simulink model "asservissement_vis_sans_fin_test"  (R2019a)
settings: Solver=VariableStepAuto  StartTime=0.0  StopTime=600000  RelTol=1e-3
model workspace (MAT data in the model file):
  Cx = 0.84
  S = 0.005625
libraries: fl_lib x14, nesl_utility x7, ee_lib x4, shared3dof x1, simulink x1, dspswit3 x1, sdl_lib x1
settings Model: Creator=Paul  LastModifiedBy=Paul

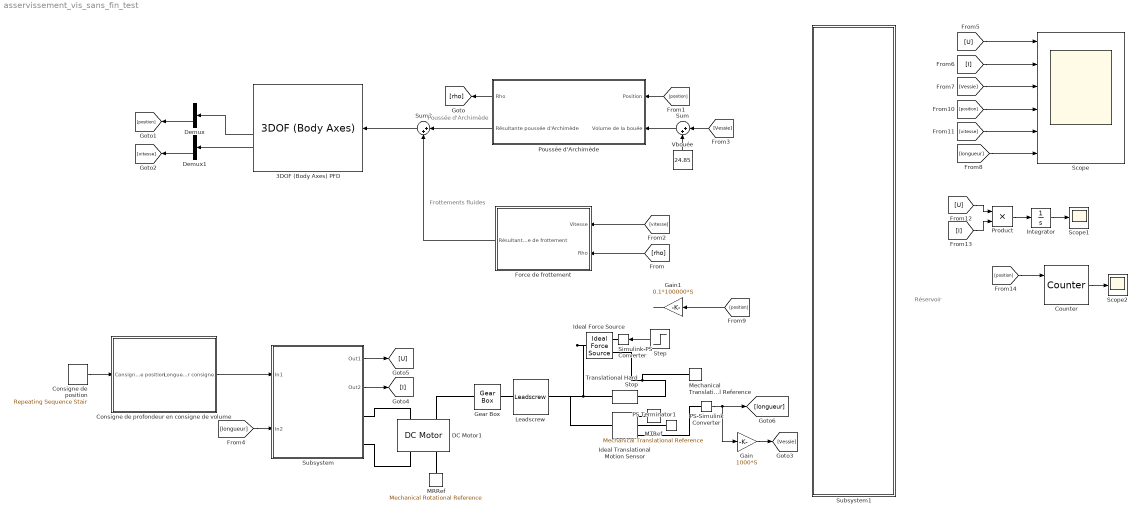
== system asservissement_vis_sans_fin_test ==
  note: Poussée d'Archimède
  note: Réservoir
  note: Frottements fluides
  "3DOF (Body Axes) PFD " : shared3dof/3DOF (Body Axes)  units=Metric (MKS)  mtype=Fixed  v_ini=0  theta_ini=0  alpha_ini=0  pos_ini=[0 0]  q_ini=0  mass=26  mass_e=0.5  mass_f=3.0  Iyy=1.0  Iyy_e=0.5  Iyy_f=3.0  g_in=Internal  g=9.81  vre_flag=on  abi_flag=off  aMode=0  vel_statename=''  theta_statename=''  pos_statename=''  q_statename=''  mass_statename=''
      settings: SourceProductName=Aerospace Blockset  SourceProductBaseCode=AE
  "Consigne de position " : simulink/Sources/Repeating Sequence Stair  OutValues=[0 1000 1000 1000 4000 0].'  tsamp=100000  OutMin=[]  OutMax=[]  OutDataTypeStr=double  OutputDataTypeScalingMode=double  OutDataType=fixdt(0,8)  ConRadixGroup=Best Precision: Vector-wise  OutScaling=2^-12
  Consigne de profondeur en consigne de volume : Subsystem
  Counter : dspswit3/Counter  Direction=Up  CountEvent=Falling edge  CounterSize=User defined  MaxCount=255  InitialCount=0  Output=Count  HitValue=32  ResetInput=on  SamplesPerFrame=1  Ts=1  CntDtype=double  HitDtype=Logical
  DC Motor1 : ee_lib/Electromechanical/Brushed Motors/DC Motor  parameterization=3  Ra=10 Ohm  La=0.0001 H  emf_or_torque=1  Kv=0.1 V/rpm  Ki=6.876e-4 N*m/A  T_stall=0.24e-3 N*m  w_max=5000 rpm  w_rated=4000 rpm  P_rated=400 W  V_rated=12 V  J=2000 g*cm^2  lam_param=1  lam=1e-6 N*m/(rad/s)  i_noload=0 A  V_i_noload=1.5 V  speed0=0 rpm  alpha=3.93e-3 1/K  Tmeas=25 degC  thermal_mass=100 J/K  initial_temperature=25 degC
      settings: SourceProductName=Simscape Electrical
  Demux : Demux  Outputs=2
  Demux1 : Demux  Outputs=2
  Force de frottement : Subsystem
  Gain : Gain  Gain=1000*S
  Gain1 : Gain  Gain=0.1*100000*S
  Gear Box : fl_lib/Mechanical/Mechanisms/Gear Box  ratio=50  t_in_specify=off  t_in_priority=None  t_in=0 N*m  t_in_nominal_specify=off  t_in_nominal_unit=N*m  t_in_nominal_value=1  t_out_specify=off  t_out_priority=None  t_out=0 N*m  t_out_nominal_specify=off  t_out_nominal_unit=N*m  t_out_nominal_value=1
  Ideal Force Source : fl_lib/Mechanical/Mechanical Sources/Ideal Force Source
  Ideal Translational Motion Sensor : fl_lib/Mechanical/Mechanical Sensors/Ideal Translational Motion Sensor  Tag=Factory Generic  offset=0.08 m
  Integrator : Integrator
  Leadscrew : sdl_lib/Gears/Rotational- Translational/Leadscrew  Lead=0.015 m  helix_type=1  friction_model=2  friction_parameterization=2  lambda=15 deg  alpha=14.5 deg  fr_coeff=0.08  eff_sn=0.9  eff_ns=0  mu_visc=0 N*m/(rad/s)  pwr_thr=0.001 W  temperature_TLU=[280, 300, 320] K  efficiency_sn_TLU=[.75, .65, .6]  efficiency_ns_TLU=[.5, .45, .4]  thermal_mass=50 J/K  T_init=300 K
      settings: SourceProductName=Simscape Driveline  SourceProductBaseCode=LD
  MRRef : fl_lib/Mechanical/Rotational Elements/Mechanical Rotational Reference
  MTRef : fl_lib/Mechanical/Translational Elements/Mechanical Translational Reference  Tag=Factory Generic
  Mechanical Translational Reference : fl_lib/Mechanical/Translational Elements/Mechanical Translational Reference
  PS Terminator1 : fl_lib/Physical Signals/Sinks/PS Terminator
      settings: SourceProductName=Simscape
  PS-Simulink Converter : nesl_utility/PS-Simulink Converter  PhysicalDomain=network_engine_domain  SubClassName=ps_output  LeftPortType=input  RightPortType=output  PseudoPeriodic=off  Frequencies=[]  Unit=1  AffineConversion=off
  Poussée d'Archimède : Subsystem
  Product : Product
  Scope : Scope  NumInputPorts=6
  Scope1 : Scope
  Scope2 : Scope
  Simulink-PS Converter : nesl_utility/Simulink-PS Converter  PhysicalDomain=network_engine_domain  SubClassName=ps_input  LeftPortType=input  RightPortType=output  PseudoPeriodic=off  Frequencies=[]  NoiseDistribution=none  NoiseParameters=[]  Unit=N  AffineConversion=off  FilteringAndDerivatives=provide  SimscapeFilterOrder=1  InputFilterTimeConstant=0.001  UdotUserProvided=0
  Step : Step  Time=490000  After=0  SampleTime=0
  Subsystem : Subsystem
  Subsystem1 : Subsystem
      mask Display: image('D:\Paul\Documents\TIPE\matlab\Les+flotteurs+Argo2.jpg');
  Sum : Sum  Inputs=|++
  Sum3 : Sum  Inputs=|++
  Translational Hard Stop : fl_lib/Mechanical/Translational Elements/Translational Hard Stop  upper_bnd=0.1 m  lower_bnd=-0.1 m  stiff_up=1e6 N/m  stiff_low=1e6 N/m  D_up=150 N/(m/s)  D_low=150 N/(m/s)  model=simscape.enum.hardstop.smooth  transition=0.1 mm  v_specify=off  v_priority=None  v=0 m/s  v_nominal_specify=off  v_nominal_unit=m/s  v_nominal_value=1  f_specify=off  f_priority=None  f=0 N  f_nominal_specify=off  f_nominal_unit=N  f_nominal_value=1  x_specify=off  x_priority=High  x=0 m  x_nominal_specify=off  x_nominal_unit=m  x_nominal_value=1
  Vbouée : Constant  Value=24.85
  wires:
  Force de frottement/1(Résultante force de frottement) -> Sum3/2
  [rho] -> Force de frottement/2(Rho)
  [U] -> Product/1
  Vbouée/1 -> Sum/2
  [position] -> Scope/4
  Demux/2 -> [position]
  [Vessie] -> Sum/1
  [I] -> Scope/2
  "3DOF (Body Axes) PFD "/5 -> Demux1/1
  "3DOF (Body Axes) PFD "/4 -> Demux/1
  [vitesse] -> Scope/5
  Demux1/2 -> [vitesse]
  Product/1 -> Integrator/1
  Poussée d'Archimède/2(Résultante poussée d'Archimède) -> Sum3/1
  [vitesse] -> Force de frottement/1(Vitesse)
  [Vessie] -> Scope/3
  [position] -> Counter/1
  [U] -> Scope/1
  Poussée d'Archimède/1("Rho ") -> [rho]
  [position] -> Poussée d'Archimède/1(Position)
  Integrator/1 -> Scope1/1
  Sum3/1 -> "3DOF (Body Axes) PFD "/2
  [I] -> Product/2
  Sum/1 -> Poussée d'Archimède/2(Volume de la bouée)
  Counter/1 -> Scope2/1
  PS-Simulink Converter/1 -> [longueur], Gain/1
  Consigne de profondeur en consigne de volume/1(Longueur consigne) -> Subsystem/1(In1)
  "Consigne de position "/1 -> Consigne de profondeur en consigne de volume/1(Consigne de position)
  Gain/1 -> [Vessie]
  [longueur] -> Subsystem/2(In2)
  Subsystem/1(Out1) -> [U]
  Subsystem/2(Out2) -> [I]
  [longueur] -> Scope/6
  Gain1/1 -> ?
  [position] -> Gain1/1
  Step/1 -> Simulink-PS Converter/1
  connections:
  DC Motor1/RConn2 -- MRRef/LConn1
  Gear Box/RConn1 -- Leadscrew/LConn1
  Gear Box/LConn1 -- DC Motor1/LConn2
  Ideal Force Source/LConn1 -- Translational Hard Stop/LConn1 -- Leadscrew/RConn1 -- Ideal Translational Motion Sensor/LConn1
  DC Motor1/LConn1 -- Subsystem/RConn1
  DC Motor1/RConn1 -- Subsystem/RConn2
  Ideal Force Source/RConn2 -- Translational Hard Stop/RConn1 -- Mechanical Translational Reference/LConn1
  PS Terminator1/LConn1 -- Ideal Translational Motion Sensor/RConn2
  Ideal Translational Motion Sensor/RConn3 -- PS-Simulink Converter/LConn1
  MTRef/LConn1 -- Ideal Translational Motion Sensor/RConn1
  Simulink-PS Converter/RConn1 -- Ideal Force Source/RConn1

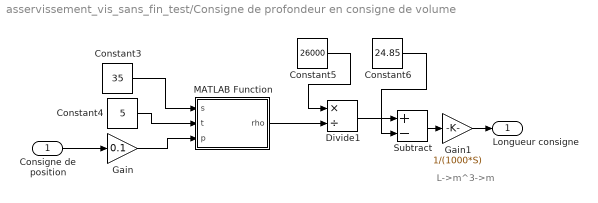
== system asservissement_vis_sans_fin_test/Consigne de profondeur en consigne de volume ==
  note: L->m^3->m
  Consigne de position : Inport
  Constant3 : Constant  Value=35
  Constant4 : Constant  Value=5
  Constant5 : Constant  Value=26000
  Constant6 : Constant  Value=24.85
  Divide1 : Product  Inputs=*/
  Gain : Gain  Gain=0.1
  Gain1 : Gain  Gain=1/(1000*S)
  MATLAB Function : MATLAB Function  TreatAsAtomicUnit=on
  Subtract : Sum  Inputs=+-
  Longueur consigne : Outport
  wires:
  Constant4/1 -> MATLAB Function/2(t)
  Divide1/1 -> Subtract/1
  Gain/1 -> MATLAB Function/3(p)
  Constant5/1 -> Divide1/1
  MATLAB Function/1(rho) -> Divide1/2
  Constant6/1 -> Subtract/2
  Constant3/1 -> MATLAB Function/1(s)
  Consigne de position/1 -> Gain/1
  Subtract/1 -> Gain1/1
  Gain1/1 -> Longueur consigne/1

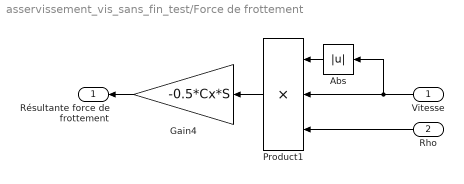
== system asservissement_vis_sans_fin_test/Force de frottement ==
  Vitesse : Inport
  Rho : Inport  Port=2
  Abs : Abs
  Gain4 : Gain  Gain=-0.5*Cx*S
  Product1 : Product  Inputs=3
  Résultante force de frottement : Outport
  wires:
  Product1/1 -> Gain4/1
  Abs/1 -> Product1/1
  Gain4/1 -> Résultante force de frottement/1
  Rho/1 -> Product1/3
  Vitesse/1 -> Abs/1, Product1/2

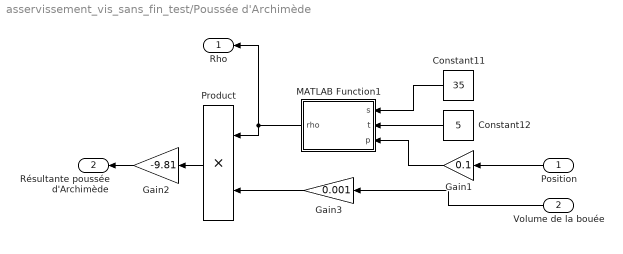
== system asservissement_vis_sans_fin_test/Poussée d'Archimède ==
  Position : Inport
  Volume de la bouée : Inport  Port=2
  Constant11 : Constant  Value=35
  Constant12 : Constant  Value=5
  Gain1 : Gain  Gain=0.1
  Gain2 : Gain  Gain=-9.81
  Gain3 : Gain  Gain=0.001
  MATLAB Function1 : MATLAB Function  TreatAsAtomicUnit=on
  Product : Product
  "Rho " : Outport
  Résultante poussée d'Archimède : Outport  Port=2
  wires:
  Position/1 -> Gain1/1
  Constant11/1 -> MATLAB Function1/1(s)
  MATLAB Function1/1(rho) -> "Rho "/1, Product/1
  Gain1/1 -> MATLAB Function1/3(p)
  Product/1 -> Gain2/1
  Constant12/1 -> MATLAB Function1/2(t)
  Gain3/1 -> Product/2
  Volume de la bouée/1 -> Gain3/1
  Gain2/1 -> Résultante poussée d'Archimède/1

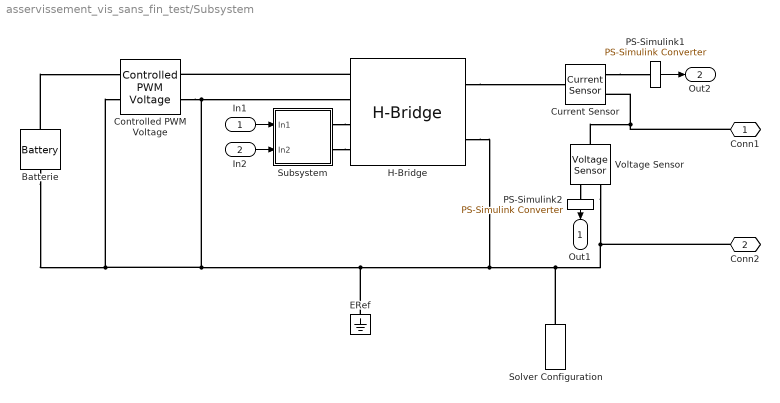
== system asservissement_vis_sans_fin_test/Subsystem ==
  In1 : Inport
  In2 : Inport  Port=2
  Batterie : ee_lib/Sources/Battery  Vnom=12 V  R1=0.06 Ohm  prm_AH=2  AH=40 hr*A  V1=10.6 V  AH1=2 hr*A  prm_R2=1  R2=2e+3 Ohm  prm_dyn=1  Rp1=0.005 Ohm  tau1=30 s  Rp2=0.005 Ohm  tau2=30 s  Rp3=0.005 Ohm  tau3=30 s  Rp4=0.005 Ohm  tau4=30 s  Rp5=0.005 Ohm  tau5=30 s  prm_fade=1  N_fade=100  AH_fade=45 hr*A  R1_fade=2.02 Ohm  V1_fade=10.35 V  i_specify=off  i_priority=None  i=0 A  i_nominal_specify=off  i_nominal_unit=A  i_nominal_value=1  v_specify=off  v_priority=None  v=0 V  v_nominal_specify=off  v_nominal_unit=V  v_nominal_value=1  charge_specify=on  charge_priority=High  charge=40 hr*A  charge_nominal_specify=off  charge_nominal_unit=hr*A  charge_nominal_value=1  num_cycles_specify=off  num_cycles_priority=High  num_cycles=0  num_cycles_nominal_specify=off  num_cycles_nominal_unit=1  num_cycles_nominal_value=1  thermal_mass=30000 J/K  Tmeas=298.15 K  Vnom_T2=12 V  R1_T2=2.2 Ohm  V1_T2=11.4 V  R2_T2=2200 Ohm  Rp1_T2=0.005 Ohm  tau1_T2=30 s  Rp2_T2=0.005 Ohm  tau2_T2=30 s  Rp3_T2=0.005 Ohm  tau3_T2=30 s  Rp4_T2=0.005 Ohm  tau4_T2=30 s  Rp5_T2=0.005 Ohm  tau5_T2=30 s  Tmeas2=273.15 K  temperature_specify=off  temperature_priority=High  temperature=298.15 K  temperature_nominal_specify=off  temperature_nominal_unit=K  temperature_nominal_value=1
      settings: SourceProductName=Simscape Electrical
  Controlled PWM Voltage : ee_lib/Integrated Circuits/Controlled PWM Voltage  F=4000 Hz  TD=0 s  pulse_width_offset=0 s  pulse_min=0 s  Vmin=0 V  Vmax=5 V  Vm=5 V  pwm_or_av=2  event_type=1  sample_time=5e-6 s  u_min=0  u_max=1
      settings: SourceProductName=Simscape Electrical
  Current Sensor : fl_lib/Electrical/Electrical Sensors/Current Sensor
  ERef : fl_lib/Electrical/Electrical Elements/Electrical Reference
  H-Bridge : ee_lib/Semiconductors & Converters/Converters/H-Bridge  Venable=2.5 V  Vmax=5 V  Vreverse=2.5 V  Vbrake=2.5 V  Vm=12 V  pwm_or_av=2  discontinuous=0  freewheeling_mode=1  freewheeling_mode_disc=1  Ron=0.1 Ohm  Don=0.1 Ohm  Rload=3.38+0.1 Ohm  Lload=1e-5 H  F=4 kHz  thermal_mass=100 J/K  initial_temperature=298.15 K  Ron2=0.1 Ohm  Don2=0.05 Ohm  Tmeas=298.15 K  Tmeas2=398.15 K
      settings: SourceProductName=Simscape Electrical
  PS-Simulink1 : nesl_utility/PS-Simulink Converter  PhysicalDomain=network_engine_domain  SubClassName=ps_output  LeftPortType=input  RightPortType=output  PseudoPeriodic=off  Frequencies=[]  Unit=A  AffineConversion=off
  PS-Simulink2 : nesl_utility/PS-Simulink Converter  PhysicalDomain=network_engine_domain  SubClassName=ps_output  LeftPortType=input  RightPortType=output  PseudoPeriodic=off  Frequencies=[]  Unit=V  AffineConversion=off
  Solver Configuration : nesl_utility/Solver Configuration  PhysicalDomain=network_engine_domain  SubClassName=solver  LeftPortType=input  RightPortType=generic  Tones=[]  Harmonics=[]  SimulateNoise=off  Profile=off  UseLocalSampling=off  EnableSwitchedLinearOptims=on  FrequencyDomain=off  UseCCode=off  RelTol=0.001  AbsTol=1e-06  MinStep=1e-09  ToWorkspace=off  RevertToSquareIcSolve=off  NumHomotopyIterations=100  PhasorMode=off  PhasorModeNumHarmonics=1  DoDC=off  ResidualTolerance=1e-9  UseLocalSolver=off  LocalSolverChoice=NE_BACKWARD_EULER_ADVANCER  LocalSolverSampleTime=5e-6  DoFixedCost=off  MaxNonlinIter=4  MaxModeIter=2  LinearAlgebra=auto  EquationFormulation=NE_TIME_EF  DelaysMemoryBudget=1024  AutomaticFiltering=on  FilteringTimeConstant=0.001  PartitionStorageMethod=AS_NEEDED  PartitionMemoryBudget=1024  PartitionMethod=FAST
  Subsystem : Subsystem
  Voltage Sensor : fl_lib/Electrical/Electrical Sensors/Voltage Sensor
  Conn1 : PMIOPort  Side=Right
  Conn2 : PMIOPort  Port=2  Side=Right
  Out1 : Outport
  Out2 : Outport  Port=2
  wires:
  PS-Simulink1/1 -> Out2/1
  PS-Simulink2/1 -> Out1/1
  In1/1 -> Subsystem/1(In1)
  In2/1 -> Subsystem/2(In2)
  connections:
  Batterie/RConn1 -- Controlled PWM Voltage/LConn2 -- Controlled PWM Voltage/RConn2 -- H-Bridge/LConn2 -- H-Bridge/RConn2 -- Conn2/RConn1 -- Voltage Sensor/RConn2 -- Solver Configuration/RConn1 -- ERef/LConn1
  Current Sensor/RConn1 -- PS-Simulink1/LConn1
  H-Bridge/RConn1 -- Current Sensor/LConn1
  Voltage Sensor/LConn1 -- Conn1/RConn1 -- Current Sensor/RConn2
  H-Bridge/LConn1 -- Controlled PWM Voltage/RConn1
  Batterie/LConn1 -- Controlled PWM Voltage/LConn1
  Voltage Sensor/RConn1 -- PS-Simulink2/LConn1
  Subsystem/RConn1 -- H-Bridge/LConn3
  Subsystem/RConn2 -- H-Bridge/LConn4

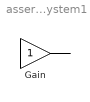
== system asservissement_vis_sans_fin_test/Subsystem1 ==
  Gain : Gain
  wires:
  ? -> Gain/1
  Gain/1 -> ?

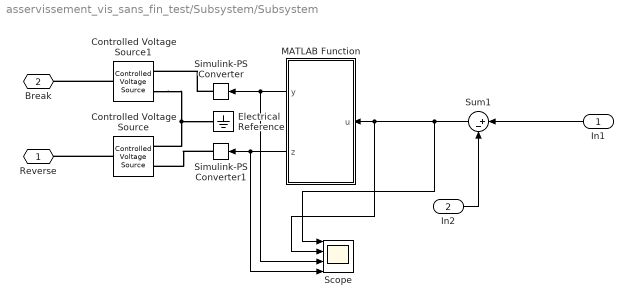
== system asservissement_vis_sans_fin_test/Subsystem/Subsystem ==
  In1 : Inport
  In2 : Inport  Port=2
  Controlled Voltage Source : fl_lib/Electrical/Electrical Sources/Controlled Voltage Source
  Controlled Voltage Source1 : fl_lib/Electrical/Electrical Sources/Controlled Voltage Source
  Electrical Reference : fl_lib/Electrical/Electrical Elements/Electrical Reference
  MATLAB Function : MATLAB Function  TreatAsAtomicUnit=on
  Scope : Scope  NumInputPorts=4
  Simulink-PS Converter : nesl_utility/Simulink-PS Converter  PhysicalDomain=network_engine_domain  SubClassName=ps_input  LeftPortType=input  RightPortType=output  PseudoPeriodic=off  Frequencies=[]  NoiseDistribution=none  NoiseParameters=[]  Unit=1  AffineConversion=off  FilteringAndDerivatives=provide  SimscapeFilterOrder=1  InputFilterTimeConstant=0.001  UdotUserProvided=0
  Simulink-PS Converter1 : nesl_utility/Simulink-PS Converter  PhysicalDomain=network_engine_domain  SubClassName=ps_input  LeftPortType=input  RightPortType=output  PseudoPeriodic=off  Frequencies=[]  NoiseDistribution=none  NoiseParameters=[]  Unit=1  AffineConversion=off  FilteringAndDerivatives=provide  SimscapeFilterOrder=1  InputFilterTimeConstant=0.001  UdotUserProvided=0
  Sum1 : Sum  Inputs=|+-
  Reverse : PMIOPort  Side=Right
  Break : PMIOPort  Port=2  Side=Right
  wires:
  In1/1 -> Sum1/1
  MATLAB Function/1(y) -> Scope/3, Simulink-PS Converter/1
  MATLAB Function/2(z) -> Scope/4, Simulink-PS Converter1/1
  In2/1 -> Sum1/2
  Sum1/1 -> Scope/2, MATLAB Function/1(u), Scope/1
  connections:
  Controlled Voltage Source1/RConn2 -- Controlled Voltage Source/RConn2 -- Electrical Reference/LConn1
  Simulink-PS Converter/RConn1 -- Controlled Voltage Source1/RConn1
  Simulink-PS Converter1/RConn1 -- Controlled Voltage Source/RConn1
  Controlled Voltage Source/LConn1 -- Reverse/RConn1
  Controlled Voltage Source1/LConn1 -- Break/RConn1

== matlab function asservissement_vis_sans_fin_test/Poussée d'Archimède/MATLAB Function1 ==
  data: s input; rho output; t input; p input
function rho=ies80(s,t,p)

% 
% International Equation of State of sea water : rho=ies80(s,t,p)
%   rho  density     (kg/m3)
%    s   salinity
%    t   temperature (°C)
%    p   pressure    (bars)
%
%    rho,s,t,p can be vector or matrix
%
%    rho=ies80(s,t) use p=0
%
%-----------------------------------
% Olivier Le Calvé 
% E-mail : lecalve@isitv.univ-tln.fr
%-----------------------------------

r0_coef=[999.842594,6.793952e-2,-9.09529e-3,1.001685e-4,-1.120083e-6,...
         6.536332e-9,8.24493e-1,-4.0899e-3,7.6438e-5,-8.2467e-7,...
         5.3875e-9,-5.72466e-3,1.0227e-4,-1.6546e-6,4.8314e-4];

r0=polyval(r0_coef(6:-1:1),t)+...
   polyval(r0_coef(11:-1:7),t).*s+...
   polyval(r0_coef(14:-1:12),t).*s.^1.5+...
   r0_coef(15)*s.^2;

if nargin==3

K_coef=[19652.21,148.4206,-2.327105,1.360447e-2,-5.155288e-5,3.239908,...
        1.43713e-3,1.16092e-4,-5.77905e-7,8.50935e-5,...
        -6.12293e-6,5.2787e-8,54.6746,-0.603459,1.09987e-2,...
        -6.1670e-5,7.944e-2,1.6483e-2,-5.3009e-4,2.2838e-3,...
        -1.0981e-5,-1.6078e-6,1.91075e-4,-9.9348e-7,...
        2.0816e-8,9.1697e-10];

K=polyval(K_coef(5:-1:1),t)+...
  polyval(K_coef(9:-1:6),t).*p+...
  polyval(K_coef(12:-1:10),t).*p.^2+...
  polyval(K_coef(16:-1:13),t).*s+...
  polyval(K_coef(19:-1:17),t).*s.^1.5+...
  polyval(K_coef(22:-1:20),t).*p.*s+...
  K_coef(23)*p.*s.^1.5+...
  polyval(K_coef(26:-1:24),t).*p.^2.*s;
  
rho=r0./(1-p./K);

else

rho=r0;

end

== matlab function asservissement_vis_sans_fin_test/Consigne de profondeur en consigne de volume/MATLAB Function ==
  data: s input; rho output; t input; p input
function rho=ies80(s,t,p)

% 
% International Equation of State of sea water : rho=ies80(s,t,p)
%   rho  density     (kg/m3)
%    s   salinity
%    t   temperature (°C)
%    p   pressure    (bars)
%
%    rho,s,t,p can be vector or matrix
%
%    rho=ies80(s,t) use p=0
%
%-----------------------------------
% Olivier Le Calvé 
% E-mail : lecalve@isitv.univ-tln.fr
%-----------------------------------

r0_coef=[999.842594,6.793952e-2,-9.09529e-3,1.001685e-4,-1.120083e-6,...
         6.536332e-9,8.24493e-1,-4.0899e-3,7.6438e-5,-8.2467e-7,...
         5.3875e-9,-5.72466e-3,1.0227e-4,-1.6546e-6,4.8314e-4];

r0=polyval(r0_coef(6:-1:1),t)+...
   polyval(r0_coef(11:-1:7),t).*s+...
   polyval(r0_coef(14:-1:12),t).*s.^1.5+...
   r0_coef(15)*s.^2;

if nargin==3

K_coef=[19652.21,148.4206,-2.327105,1.360447e-2,-5.155288e-5,3.239908,...
        1.43713e-3,1.16092e-4,-5.77905e-7,8.50935e-5,...
        -6.12293e-6,5.2787e-8,54.6746,-0.603459,1.09987e-2,...
        -6.1670e-5,7.944e-2,1.6483e-2,-5.3009e-4,2.2838e-3,...
        -1.0981e-5,-1.6078e-6,1.91075e-4,-9.9348e-7,...
        2.0816e-8,9.1697e-10];

K=polyval(K_coef(5:-1:1),t)+...
  polyval(K_coef(9:-1:6),t).*p+...
  polyval(K_coef(12:-1:10),t).*p.^2+...
  polyval(K_coef(16:-1:13),t).*s+...
  polyval(K_coef(19:-1:17),t).*s.^1.5+...
  polyval(K_coef(22:-1:20),t).*p.*s+...
  K_coef(23)*p.*s.^1.5+...
  polyval(K_coef(26:-1:24),t).*p.^2.*s;
  
rho=r0./(1-p./K);

else

rho=r0;

end

== matlab function asservissement_vis_sans_fin_test/Subsystem/Subsystem/MATLAB Function ==
  data: u input; y output; z output
function [y, z] = controle(u)
y=0;
z=0;
if (u>-0.001)&& (u<0.001)
    y=3.5;
    z=0;
    
elseif (u<-0.001) 
    z=3.5;
    y=0;
elseif u>0.001
    z=0;
    y=0;
end
end
